simulink model "three_chessclock"  (R2018b)
settings: Solver=FixedStepDiscrete  StartTime=0.0  StopTime=inf  FixedStep=0.1  RelTol=1e-3  EnableMultiTasking=on
settings Model: EnablePacing=on  PacingRate=10  Creator=Sjoerd  LastModifiedBy=svdh
settings SolverCC: AutoInsertRateTranBlk=on
settings DataIOCC: LimitDataPoints=on
settings OptimizationCC: LifeSpan=inf
settings DebuggingCC: AllowSymbolicDim=off  SFUnexpectedBacktrackingDiag=warning  SFNoUnconditionalDefaultTransitionDiag=warning  SFExecutionAtInitializationDiag=none
settings SFSimCC: SimUseLocalCustomCode=off
settings RTWCC: RTWUseLocalCustomCode=off
settings CodeAppCC: StateflowObjectComments=on
settings GRTTargetCC: TargetLangStandard=C89/C90 (ANSI)  GeneratePreprocessorConditionals=Disable all
settings ConfigComp: CovMetricSettings=dw  CovHtmlReporting=on  CovSaveCumulativeToWorkspaceVar=on  CovSaveSingleToWorkspaceVar=on  CovShowResultsExplorer=off  CovExternalEMLEnable=off  CovSFcnEnable=off

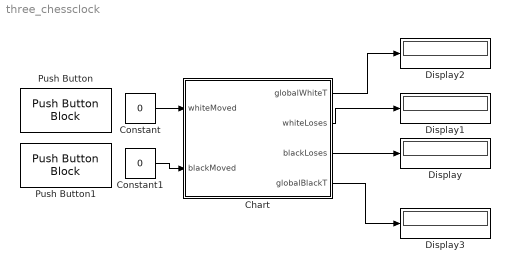
== system three_chessclock ==
  Chart : Stateflow chart  TreatAsAtomicUnit=on
  Constant : Constant  Value=0
  Constant1 : Constant  Value=0
  Display{,1..3} (4 alike) : Display
  Push Button : PushButtonBlock  WebBlockId=9  ButtonText=whiteMoved
  Push Button1 : PushButtonBlock  WebBlockId=11  ButtonText=blackMoved
  wires:
  Constant/1 -> Chart/1(whiteMoved)
  Constant1/1 -> Chart/2(blackMoved)
  Chart/2(whiteLoses) -> Display1/1
  Chart/3(blackLoses) -> Display/1
  Chart/1(globalWhiteT) -> Display2/1
  Chart/4(globalBlackT) -> Display3/1

== stateflow chart three_chessclock/Chart ==
  state White
    state white1 [parallel]
      settings: executionOrder=1
      state localTick
      state localTock
        entry: localWhiteT = localWhiteT - 1
      state globalTick
      state globalTock
        entry: globalWhiteT = globalWhiteT -1
      state Boom
        whiteLoses = 1
      (default) -> White.white1.localTick : {localWhiteT = 10}
      White.white1.localTick -> White.white1.localTock : after(1,sec)
      White.white1.localTock -> White.white1.localTick [order 2] : [localWhiteT > 0]
      White.white1.localTock -> White.white1.globalTick [order 1] : [localWhiteT == 0]
      White.white1.globalTick -> White.white1.globalTock : after(1,sec)
      White.white1.globalTock -> White.white1.globalTick [order 1] : [globalWhiteT > 0]
      White.white1.globalTock -> White.white1.Boom [order 2] : [globalWhiteT == 0]
    state movechecker [parallel]
      settings: executionOrder=2
      state manymoves
        entry:
        globalWhiteT = globalWhiteT + (15*60)
        globalBlackT = globalBlackT + (15*60)
      state fewmoves
      (default) -> fewmoves
      fewmoves -> manymoves : [moves == 40]
  state Black
    state localTick
    state localTock
      entry: localBlackT = localBlackT - 1
    state globalTick
    state globalTock
      entry: globalBlackT = globalBlackT -1
    state Boom
      blackLoses = 1
    (default) -> Black.localTick : {localBlackT = 10}
    Black.localTick -> Black.localTock : after(1,sec)
    Black.localTock -> Black.localTick [order 2] : [localBlackT > 0]
    Black.localTock -> Black.globalTick [order 1] : [localBlackT == 0]
    Black.globalTick -> Black.globalTock : after(1,sec)
    Black.globalTock -> Black.globalTick [order 1] : [globalBlackT > 0]
    Black.globalTock -> Black.Boom [order 2] : [globalBlackT == 0]
  (default) -> White [order 1] : {globalWhiteT = 60; whiteLoses = 0;globalBlackT = 60; blackLoses = 0; moves = 0 }
  White -> Black : [whiteMoved == 1]{globalWhiteT = globalWhiteT + 15}
  (default) -> White [order 2] : [blackMoved == 1]{globalBlackT = globalBlackT + 15; moves = moves + 1
      | }
  data: globalWhiteT output; whiteLoses output; blackLoses output; whiteMoved input; blackMoved input; localBlackT local; localWhiteT local; globalBlackT output; moves local
